simulink model "especiesMIMO"  (R2022a)
settings: Solver=VariableStepAuto  StartTime=0  StopTime=10000  FixedStep=4.53134094146028  RelTol=1e-3
model workspace (MAT data in the model file):
  a = 0.2586
  b = 0.0203
  c = 0.0574
  d = 0.0097
  m = 0.0571
  n = 0.0048
  u = 0.05
  x0 = 0.6765
  y0 = 5.5828
undefined symbols (not defined in the file): K, sigbuilder_block, unom
settings Model: Creator=LuisaToro  LastModifiedBy=LuisaToro
settings DataIOCC: SaveFormat=Array  OutputTimes=tout
settings DebuggingCC: UnconnectedInputMsg=warning  UnconnectedOutputMsg=warning  UnconnectedLineMsg=warning
settings RTWCC: DLArmComputeVersion=19.05

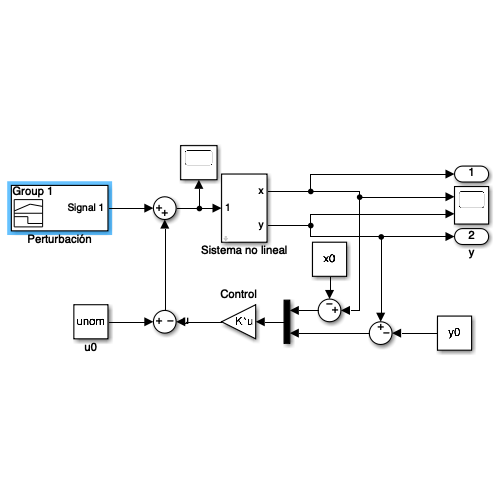
[thumbnail: Simulink's stored preview of the top-level diagram]
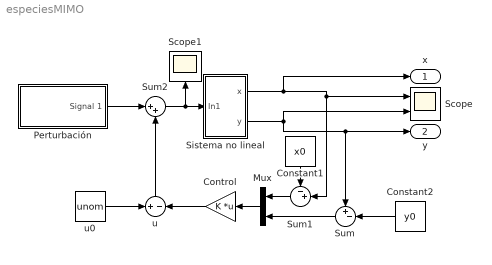
== system especiesMIMO ==
  Constant1 : Constant  Value=x0  VectorParams1D=off
  Constant2 : Constant  Value=y0  VectorParams1D=off
  Control : Gain  Gain=K  Multiplication=Matrix(K*u)
  Mux : Mux  Inputs=2
  Perturbación : Subsystem  Tag=STV Subsys  LoadFcn=sigbuilder_block('load');  StartFcn=sigbuilder_block('start');  StopFcn=sigbuilder_block('stop');  ClipboardFcn=sigbuilder_block('clipboard');  mask(Sigbuilder block){tuvar=[0:10]}
      mask help: Simulink:masks:SigbuilderBlock_MD
      mask init:
      | if ~strcmp(get_param(bdroot(gcbh),'SimulationStatus'),'stopped') tuvar = sigbuilder_block('maskInit'); end
      settings: CopyFcn=sigbuilder_block('copy');  DeleteFcn=sigbuilder_block('delete');  ModelCloseFcn=sigbuilder_block('modelClose');  PreSaveFcn=sigbuilder_block('preSave');  PauseFcn=sigbuilder_block('pause');  ContinueFcn=sigbuilder_block('continue');  NameChangeFcn=sigbuilder_block('namechange');  OpenFcn=sigbuilder_block('open',[437.6 199.2 550.4 400 ]);  CloseFcn=sigbuilder_block('close');
      mask Display: plot(0, 0, 100, 100,[2, 2, 32, 32, 2], [68, 8, 8, 68, 68],[32, 2], [38, 38], [32, 19, 2],[53, 60, 44], [32, 17, 17, 2],[16, 16, 31, 31]);txt = getActiveGroup(gcbh);text(2, 100, txt,'verticalAlignment', 'top');
  Scope : Scope  NumInputPorts=2
  Scope1 : Scope
  Sistema no lineal : Subsystem  mask{a=a, b=b, c=c, d=d, m=m, n=n, x0=x0, y0=y0}
  Sum : Sum  Inputs=+-|
  Sum1 : Sum  Inputs=-+|
  Sum2 : Sum  Inputs=|++
  u : Sum  Inputs=+-
  u0 : Constant  Value=unom
  x : Outport
  y : Outport  Port=2
  wires:
  Sistema no lineal/1(x) -> Sum1/2, Scope/1, x/1
  Sistema no lineal/2(y) -> Sum/1, y/1, Scope/2
  Perturbación/1(Signal 1) -> Sum2/1
  Sum2/1 -> Sistema no lineal/1(In1), Scope1/1
  u/1 -> Sum2/2
  Mux/1 -> Control/1
  Sum1/1 -> Mux/1
  Constant1/1 -> Sum1/1
  Sum/1 -> Mux/2
  Constant2/1 -> Sum/2
  u0/1 -> u/1
  Control/1 -> u/2

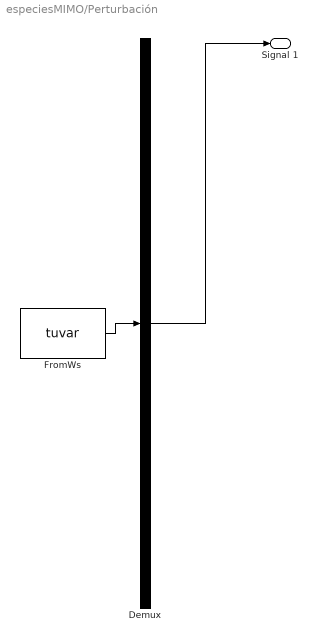
== system especiesMIMO/Perturbación ==
  Demux : Demux  Tag=STV Demux  Outputs=1
      settings: DisplayOption=none
  FromWs : FromWorkspace  Tag=STV FromWs  VariableName=tuvar
      SigBuilderData=|
      | common.afterFinalStr = 'Extrapolate'
      | common.sampleTime = 0
      | dataSet.timeRange = [0 10000]
      | dataSet.name = 'Group 1'
      | sbobj.Groups.Name = 'Group 1'
      | sbobj.Groups.Signals.Name = 'Signal 1'
      | sbobj.Groups.Signals.XData = [0 5000 5000 10000]
      | sbobj.Groups.Signals.YData = [0 0 0.1 0.1]
      | sbobj.Groups.TimeRange = [0 10000]
  Signal 1 : Outport  Tag=STV Outport
  wires:
  Demux/1 -> Signal 1/1
  FromWs/1 -> Demux/1

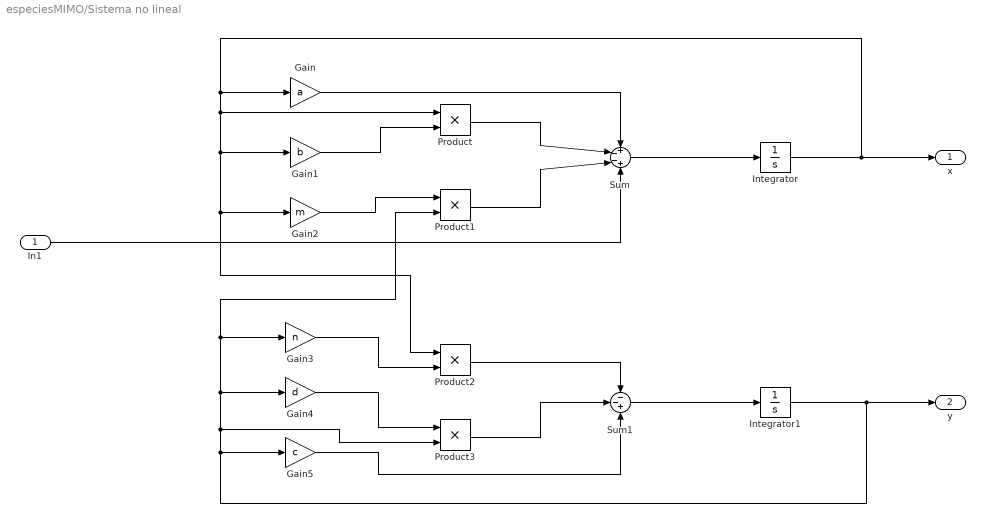
== system especiesMIMO/Sistema no lineal ==
  In1 : Inport
  Gain : Gain  Gain=a
  Gain1 : Gain  Gain=b
  Gain2 : Gain  Gain=m
  Gain3 : Gain  Gain=n
  Gain4 : Gain  Gain=d
  Gain5 : Gain  Gain=c
  Integrator : Integrator  InitialCondition=x0  LimitOutput=on  LowerSaturationLimit=0
  Integrator1 : Integrator  InitialCondition=y0  LimitOutput=on  LowerSaturationLimit=0
  Product{,1..3} (4 alike) : Product
  Sum : Sum  Inputs=+--+
  Sum1 : Sum  Inputs=--+
  x : Outport
  y : Outport  Port=2
  wires:
  Product2/1 -> Sum1/1
  Gain/1 -> Sum/1
  Product1/1 -> Sum/3
  Gain1/1 -> Product/2
  Product3/1 -> Sum1/2
  Sum1/1 -> Integrator1/1
  Gain3/1 -> Product2/2
  Product/1 -> Sum/2
  Integrator/1 -> x/1, Product/1, Product2/1, Gain2/1, Gain1/1, Gain/1
  Sum/1 -> Integrator/1
  Gain4/1 -> Product3/1
  In1/1 -> Sum/4
  Integrator1/1 -> y/1, Product3/2, Product1/2, Gain3/1, Gain4/1, Gain5/1
  Gain2/1 -> Product1/1
  Gain5/1 -> Sum1/3
